simulink model "E3_QSM"  (R2025a)
settings: Solver=ode4  StartTime=0.0  StopTime=15  FixedStep=0.002  RelTol=1e-3  EnableMultiTasking=on
undefined symbols (not defined in the file): g, Jp_cm, kt, l, mode, mp, mr, nis, out_planta_e3, p, r, ref, Rm, seq, TET, tmodel, twall, Vm, xhat
libraries: simulink x6, quarc_library x4
settings Model: ExtModeTrigDuration=10000  Creator=sebas  LastModifiedBy=sebas
settings SolverCC: AlgebraicLoopSolver=TrustRegion  PositivePriorityOrder=on  EnableFixedStepZeroCrossing=on
settings DataIOCC: ReturnWorkspaceOutputs=off
settings DebuggingCC: UnconnectedInputMsg=warning  UnconnectedOutputMsg=warning  UnconnectedLineMsg=warning  ArithmeticOperatorsInVariantConditions=warning
settings HardwareCC: ProdHWDeviceType=AMD->x86-64 (Windows64)
settings ModelReferenceCC: EnableRefExpFcnMdlSchedulingChecks=on
settings SFSimCC: SimUseLocalCustomCode=off  CustomCodeUndefinedFunction=UseInterfaceOnly
settings RTWCC: SystemTargetFile=quarc_win64.tlc  TemplateMakefile=quarc_default_tmf  RTWUseLocalCustomCode=off  Toolchain=QUARC win64 | nmake (64-bit Windows)  BuildConfiguration=Faster Runs  GPUComputeCapability=3.5  Description=QUARC Win64 Target Using Toolchain
settings CodeAppCC: StateflowObjectComments=on
settings STFCustomTargetCC: SystemTargetFile=quarc_win64.tlc  TargetLangStandard=C99 (ISO)  MultiwordLength=2048.0  DynamicStringBufferSize=256.0  ConcurrentExecutionCompliant=on  UseToolchainInfoCompliant=on
settings GRTTargetCC: ExtMode=on  ExtModeMexFile=quarc_comm  ParMdlRefBuildCompliant=off  CompOptLevelCompliant=off  CombineOutputUpdateFcns=off  MatFileLogging=off  CPPClassGenCompliant=off  GRTInterface=on
settings ConfigComp: CovMetricSettings=dswe

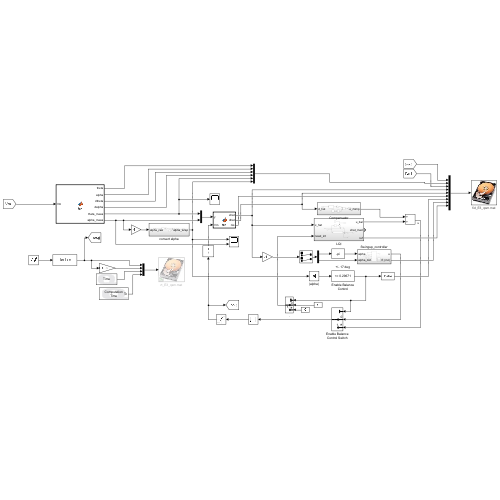
[thumbnail: Simulink's stored preview of the top-level diagram]
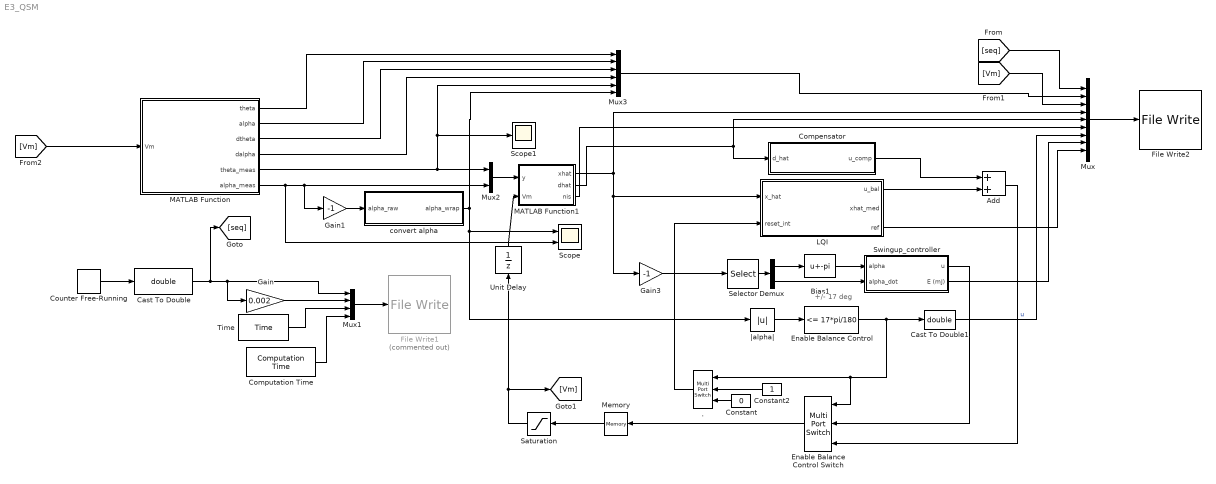
== system E3_QSM ==
  note: +/- 17 deg
  . : MultiPortSwitch  DataPortOrder=Zero-based contiguous  Inputs=2  zeroidx=on  SaturateOnIntegerOverflow=off  InputSameDT=off
  Add : Sum
  Bias1 : Bias  Bias=-pi  SaturateOnIntegerOverflow=off
  Cast To Double : DataTypeConversion  OutDataTypeStr=double  SaturateOnIntegerOverflow=off  RndMeth=Floor
  Cast To Double1 : DataTypeConversion  OutDataTypeStr=double  SaturateOnIntegerOverflow=off  RndMeth=Floor
  Compensator : Subsystem
  Computation Time : quarc_library/Sources/Time/Computation Time  sample_time=qc_get_step_size  use_model=on  use_cpu_time=off
  Constant : Constant  Value=0
  Constant2 : Constant
  Counter Free-Running : simulink/Sources/Counter Free-Running  NumBits=16  tsamp=-1
  Demux : Demux  Outputs=2
  Enable Balance Control : simulink/Logic and Bit Operations/Compare To Constant  relop=<=  const=17*pi/180  OutDataTypeStr=boolean  ZeroCross=off
  Enable Balance Control Switch : MultiPortSwitch  DataPortOrder=Zero-based contiguous  Inputs=2  zeroidx=on  SaturateOnIntegerOverflow=off  InputSameDT=off
  File Write1 : quarc_library/Sinks/To Target/File Write  Commented=on  source=Specify via dialog (do not evaluate)  file_name=rt_E3_qsm.mat  variable_name=seq,tmodel,twall,TET  decimation=1  sample_time=-1  file_format=MAT-file v.4  options=No header or footer  append=off  encoding=Default  bitrate=0
      settings: AttributesFormatString=%<file_name>  SourceProductName=QUARC Targets
  File Write2 : quarc_library/Sinks/To Target/File Write  source=Specify via dialog (do not evaluate)  file_name=fid_E3_qsm.mat  variable_name=seq,out_planta_e3,Vm,xhat.dhat,nis,mode,E,ref  decimation=1  sample_time=-1  file_format=MAT-file v.4  options=No header or footer  append=off  encoding=Default  bitrate=0
      settings: AttributesFormatString=%<file_name>  SourceProductName=QUARC Targets
  Gain : Gain  Gain=0.002
  Gain1 : Gain  Gain=-1
  Gain3 : Gain  Gain=-1
  LQI : Subsystem
  MATLAB Function : MATLAB Function  TreatAsAtomicUnit=on
  MATLAB Function1 : MATLAB Function  TreatAsAtomicUnit=on
  Memory : Memory  InheritSampleTime=on  LinearizeMemory=on  LinearizeAsDelay=on
  Mux : Mux  Inputs=9
  Mux1 : Mux
  Mux2 : Mux  Inputs=2
  Mux3 : Mux  Inputs=6
  Saturation : Saturate  UpperLimit=10  LowerLimit=-10
  Scope : Scope  NumInputPorts=2
      settings: ActiveDisplayYMinimum=-4.2429908592916838  ActiveDisplayYMaximum=6.77099119772722
  Scope1 : Scope
      settings: ActiveDisplayYMinimum=-0.93687876620115529  ActiveDisplayYMaximum=1.4676361188095872
  Selector : Selector  InputPortWidth=4  IndexOptions=Index vector (dialog)  Indices=[2 4]  OutputSizes=1
  Swingup_controller : Subsystem
  Time : quarc_library/Sources/Time/Time  time_source=Wall clock  sample_time=qc_get_step_size
  Unit Delay : UnitDelay  SampleTime=-1  HasFrameUpgradeWarning=on
  convert alpha : Subsystem
  |alpha| : Abs  SaturateOnIntegerOverflow=off
  wires:
  Computation Time/1 -> Mux1/4
  Gain/1 -> Mux1/2
  Time/1 -> Mux1/3
  Cast To Double/1 -> [seq], Mux1/1, Gain/1
  Mux1/1 -> File Write1/1
  Counter Free-Running/1 -> Cast To Double/1
  MATLAB Function1/2(dhat) -> Mux/5, Compensator/1(d_hat)
  LQI/1(u_bal) -> Add/2
  Compensator/1(u_comp) -> Add/1
  Selector/1 -> Demux/1
  |alpha|/1 -> Enable Balance Control/1
  Unit Delay/1 -> MATLAB Function1/2(Vm)
  MATLAB Function1/1(xhat) -> LQI/1(x_hat), Gain3/1, Mux/4
  Constant2/1 -> ./2
  Add/1 -> Enable Balance Control Switch/3  "u"
  Bias1/1 -> Swingup_controller/1(alpha)
  Constant/1 -> ./3
  Enable Balance Control/1 -> Cast To Double1/1, Enable Balance Control Switch/1, ./1
  Demux/2 -> Swingup_controller/2(alpha_dot)
  Demux/1 -> Bias1/1
  Swingup_controller/1(u) -> Enable Balance Control Switch/2
  Saturation/1 -> [Vm], Unit Delay/1
  Gain3/1 -> Selector/1
  ./1 -> LQI/2(reset_int)
  convert alpha/1(alpha_wrap) -> Mux3/6, |alpha|/1, Scope/1
  Mux2/1 -> MATLAB Function1/1(y)
  [seq] -> Mux/1
  MATLAB Function/3(dtheta) -> Mux3/3
  MATLAB Function/4(dalpha) -> Mux3/4
  Mux3/1 -> Mux/2
  [Vm] -> Mux/3
  MATLAB Function1/3(nis) -> Mux/6
  Swingup_controller/2(E (mJ)) -> Mux/8
  LQI/3(ref) -> Mux/9
  Mux/1 -> File Write2/1
  Cast To Double1/1 -> Mux/7
  MATLAB Function/2(alpha) -> Mux3/2
  Enable Balance Control Switch/1 -> Memory/1
  MATLAB Function/5(theta_meas) -> Mux2/1, Scope1/1, Mux3/5
  MATLAB Function/1(theta) -> Mux3/1
  [Vm] -> MATLAB Function/1(Vm)
  Memory/1 -> Saturation/1
  MATLAB Function/6(alpha_meas) -> Mux2/2, Gain1/1, Scope/2
  Gain1/1 -> convert alpha/1(alpha_raw)

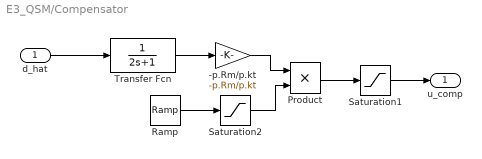
== system E3_QSM/Compensator ==
  d_hat : Inport
  -p.Rm/p.kt : Gain  Gain=-p.Rm/p.kt
  Product : Product
  Ramp : simulink/Sources/Ramp  slope=0.5  start=0  InitialOutput=0
  Saturation1 : Saturate  UpperLimit=2  LowerLimit=-2
  Saturation2 : Saturate  UpperLimit=1  LowerLimit=0
  Transfer Fcn : TransferFcn  Denominator=[2 1]
  u_comp : Outport
  wires:
  Saturation1/1 -> u_comp/1
  Transfer Fcn/1 -> -p.Rm/p.kt/1
  -p.Rm/p.kt/1 -> Product/1
  Saturation2/1 -> Product/2
  Ramp/1 -> Saturation2/1
  d_hat/1 -> Transfer Fcn/1
  Product/1 -> Saturation1/1

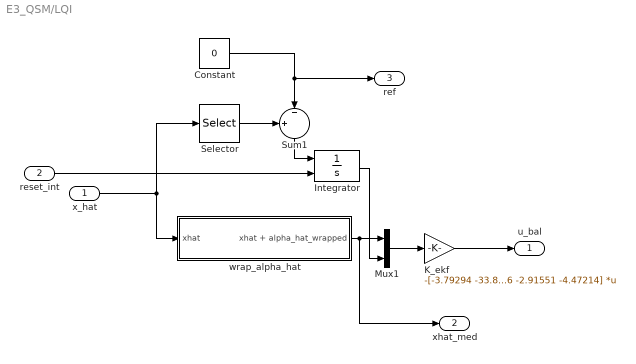
== system E3_QSM/LQI ==
  x_hat : Inport
  reset_int : Inport  Port=2
  Constant : Constant  Value=0
  Integrator : Integrator  ExternalReset=level hold  LimitOutput=on  UpperSaturationLimit=2  LowerSaturationLimit=-2
  K_ekf : Gain  Gain=-[-3.79294 -33.8988 -1.48036 -2.91551 -4.47214]  Multiplication=Matrix(K*u)
  Mux1 : Mux  Inputs=2
  Selector : Selector  InputPortWidth=4  IndexOptions=Index vector (dialog)  Indices=[1]  OutputSizes=1
  Sum1 : Sum  Inputs=+|-||
  wrap_alpha_hat : Subsystem
  u_bal : Outport
  xhat_med : Outport  Port=2
  ref : Outport  Port=3
  wires:
  Integrator/1 -> Mux1/2
  Mux1/1 -> K_ekf/1
  Constant/1 -> ref/1, Sum1/2
  Sum1/1 -> Integrator/1
  Selector/1 -> Sum1/1
  K_ekf/1 -> u_bal/1
  reset_int/1 -> Integrator/2
  x_hat/1 -> wrap_alpha_hat/1(xhat), Selector/1
  wrap_alpha_hat/1(xhat + alpha_hat_wrapped) -> xhat_med/1, Mux1/1

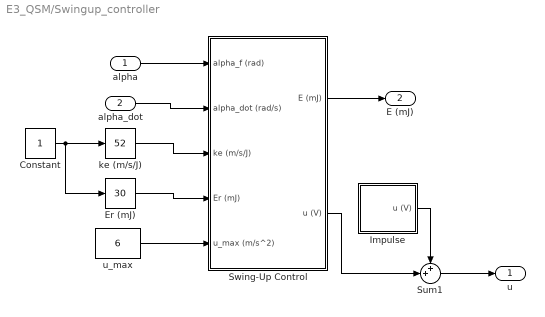
== system E3_QSM/Swingup_controller ==
  alpha : Inport
  alpha_dot : Inport  Port=2
  Constant : Constant
  Er (mJ) : simulink/Math Operations/Slider Gain  gain=30  low=0  high=100
  Impulse : Subsystem
  Sum1 : Sum  Inputs=++|
  Swing-Up Control : Subsystem
  ke (m/s/J) : simulink/Math Operations/Slider Gain  gain=52  low=0  high=100
  u_max : Constant  Value=6
  u : Outport
  E (mJ) : Outport  Port=2
  wires:
  alpha/1 -> Swing-Up Control/1(alpha_f (rad))
  Sum1/1 -> u/1
  u_max/1 -> Swing-Up Control/5(u_max (m/s^2))
  Impulse/1(u (V)) -> Sum1/1
  Swing-Up Control/1(E (mJ)) -> E (mJ)/1
  Swing-Up Control/2(u (V)) -> Sum1/2
  ke (m/s/J)/1 -> Swing-Up Control/3(ke (m/s/J))
  Constant/1 -> Er (mJ)/1, ke (m/s/J)/1
  Er (mJ)/1 -> Swing-Up Control/4(Er (mJ))
  alpha_dot/1 -> Swing-Up Control/2(alpha_dot (rad/s))

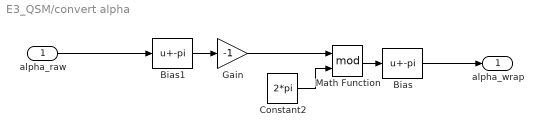
== system E3_QSM/convert alpha ==
  alpha_raw : Inport
  Bias : Bias  Bias=-pi  SaturateOnIntegerOverflow=off
  Bias1 : Bias  Bias=-pi  SaturateOnIntegerOverflow=off
  Constant2 : Constant  Value=2*pi
  Gain : Gain  Gain=-1
  Math Function : Math  Operator=mod  SignedPower=on
  alpha_wrap : Outport
  wires:
  Math Function/1 -> Bias/1
  Bias/1 -> alpha_wrap/1
  Constant2/1 -> Math Function/2
  alpha_raw/1 -> Bias1/1
  Bias1/1 -> Gain/1
  Gain/1 -> Math Function/1

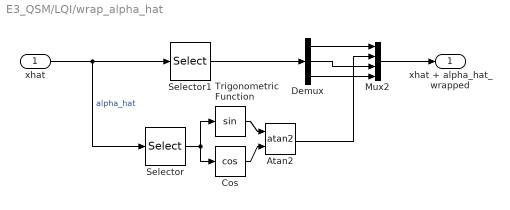
== system E3_QSM/LQI/wrap_alpha_hat ==
  xhat : Inport
  Atan2 : Trigonometry  Operator=atan2
  Cos : Trigonometry  Operator=cos
  Demux : Demux  Outputs=3
  Mux2 : Mux
  Selector : Selector  InputPortWidth=4  IndexOptions=Index vector (dialog)  Indices=[2]  OutputSizes=1
  Selector1 : Selector  InputPortWidth=4  IndexOptions=Index vector (dialog)  Indices=[1 3 4]  OutputSizes=1
  Trigonometric Function : Trigonometry
  xhat + alpha_hat_wrapped : Outport
  wires:
  Selector/1 -> Cos/1, Trigonometric Function/1
  Mux2/1 -> xhat + alpha_hat_wrapped/1
  Cos/1 -> Atan2/2
  xhat/1 -> Selector/1, Selector1/1  "alpha_hat"
  Trigonometric Function/1 -> Atan2/1
  Demux/2 -> Mux2/3
  Selector1/1 -> Demux/1
  Demux/1 -> Mux2/1
  Demux/3 -> Mux2/4
  Atan2/1 -> Mux2/2

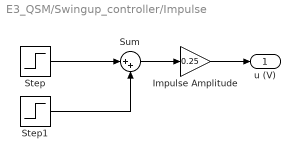
== system E3_QSM/Swingup_controller/Impulse ==
  Impulse Amplitude : Gain  Gain=0.25
  Step : Step  SampleTime=0
  Step1 : Step  Time=1.1  After=-1  SampleTime=0
  Sum : Sum  Inputs=|++
  u (V) : Outport  VectorParamsAs1DForOutWhenUnconnected=off
  wires:
  Impulse Amplitude/1 -> u (V)/1
  Sum/1 -> Impulse Amplitude/1
  Step/1 -> Sum/1
  Step1/1 -> Sum/2

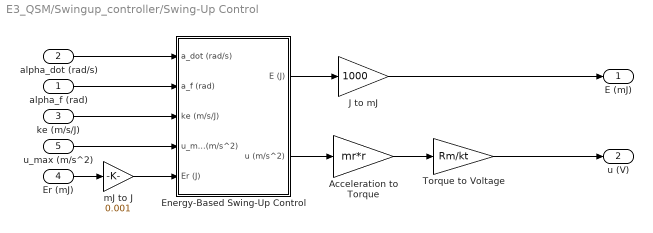
== system E3_QSM/Swingup_controller/Swing-Up Control ==
  alpha_f (rad) : Inport
  alpha_dot (rad/s) : Inport  Port=2
  ke (m/s/J) : Inport  Port=3
  Er (mJ) : Inport  Port=4
  u_max (m/s^2) : Inport  Port=5
  Acceleration to Torque : Gain  Gain=mr*r
  Energy-Based Swing-Up Control : Subsystem
  J to mJ : Gain  Gain=1000
  Torque to Voltage : Gain  Gain=Rm/kt
  mJ to J : Gain  Gain=0.001
  E (mJ) : Outport  VectorParamsAs1DForOutWhenUnconnected=off
  u (V) : Outport  Port=2  VectorParamsAs1DForOutWhenUnconnected=off
  wires:
  mJ to J/1 -> Energy-Based Swing-Up Control/5(Er (J))
  alpha_dot (rad/s)/1 -> Energy-Based Swing-Up Control/1(a_dot (rad/s))
  Torque to Voltage/1 -> u (V)/1
  J to mJ/1 -> E (mJ)/1
  Er (mJ)/1 -> mJ to J/1
  Acceleration to Torque/1 -> Torque to Voltage/1
  u_max (m/s^2)/1 -> Energy-Based Swing-Up Control/4(u_max (m/s^2))
  ke (m/s/J)/1 -> Energy-Based Swing-Up Control/3(ke (m/s/J))
  alpha_f (rad)/1 -> Energy-Based Swing-Up Control/2(a_f (rad))
  Energy-Based Swing-Up Control/1(E (J)) -> J to mJ/1
  Energy-Based Swing-Up Control/2(u (m/s^2)) -> Acceleration to Torque/1

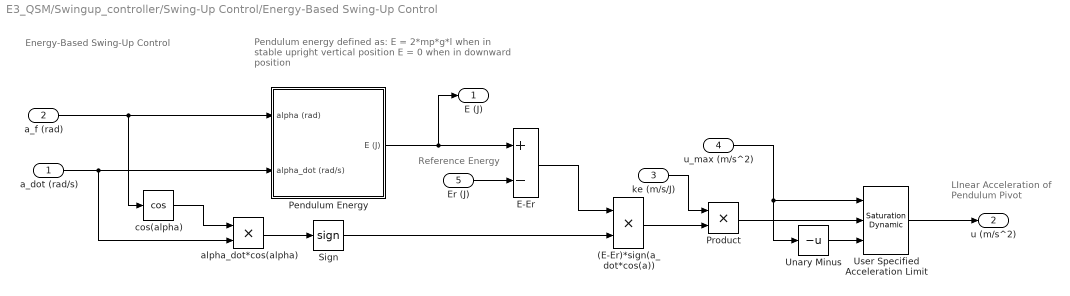
== system E3_QSM/Swingup_controller/Swing-Up Control/Energy-Based Swing-Up Control ==
  note: Pendulum energy defined as:
      | E = 2*mp*g*l when in stable upright vertical position
      | E = 0 when in downward position
  note: Reference Energy
  note: LInear Acceleration of
      | Pendulum Pivot
  note: Energy-Based Swing-Up Control
  a_dot (rad/s) : Inport
  a_f (rad) : Inport  Port=2
  ke (m/s/J) : Inport  Port=3
  u_max (m/s^2) : Inport  Port=4
  Er (J) : Inport  Port=5
  (E-Er)*sign(a_dot*cos(a)) : Product  RndMeth=Zero
  E-Er : Sum  Inputs=+-
  Pendulum Energy : Subsystem
  Product : Product  RndMeth=Zero
  Sign : Signum
  Unary Minus : UnaryMinus
  User Specified Acceleration Limit : simulink/Discontinuities/Saturation Dynamic  OutMin=[]  OutMax=[]  OutDataTypeStr=Inherit: Same as second input  OutDataType=fixdt(1, 16)  OutScaling=2^-10  DoSatur=off
  alpha_dot*cos(alpha) : Product  RndMeth=Zero
  cos(alpha) : Trigonometry  Operator=cos
  E (J) : Outport  VectorParamsAs1DForOutWhenUnconnected=off
  u (m/s^2) : Outport  Port=2  VectorParamsAs1DForOutWhenUnconnected=off
  wires:
  User Specified Acceleration Limit/1 -> u (m/s^2)/1
  Unary Minus/1 -> User Specified Acceleration Limit/3
  u_max (m/s^2)/1 -> Unary Minus/1, User Specified Acceleration Limit/1
  Product/1 -> User Specified Acceleration Limit/2
  ke (m/s/J)/1 -> Product/1
  Er (J)/1 -> E-Er/2
  (E-Er)*sign(a_dot*cos(a))/1 -> Product/2
  a_dot (rad/s)/1 -> Pendulum Energy/2(alpha_dot (rad/s)), alpha_dot*cos(alpha)/2
  Pendulum Energy/1(E (J)) -> E-Er/1, E (J)/1
  E-Er/1 -> (E-Er)*sign(a_dot*cos(a))/1
  cos(alpha)/1 -> alpha_dot*cos(alpha)/1
  alpha_dot*cos(alpha)/1 -> Sign/1
  Sign/1 -> (E-Er)*sign(a_dot*cos(a))/2
  a_f (rad)/1 -> cos(alpha)/1, Pendulum Energy/1(alpha (rad))

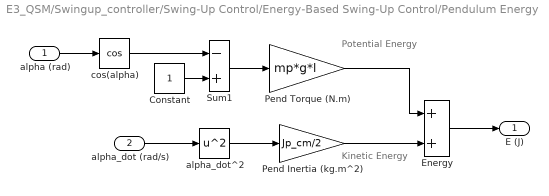
== system E3_QSM/Swingup_controller/Swing-Up Control/Energy-Based Swing-Up Control/Pendulum Energy ==
  note: Potential Energy
  note: Kinetic Energy
  alpha (rad) : Inport
  alpha_dot (rad/s) : Inport  Port=2
  Constant : Constant
  Energy : Sum  SaturateOnIntegerOverflow=on
  Pend Inertia (kg.m^2) : Gain  Gain=Jp_cm/2
  Pend Torque (N.m) : Gain  Gain=mp*g*l
  Sum1 : Sum  Inputs=-+  SaturateOnIntegerOverflow=on
  alpha_dot^2 : Math  Operator=square  SignedPower=on
  cos(alpha) : Trigonometry  Operator=cos
  E (J) : Outport  VectorParamsAs1DForOutWhenUnconnected=off
  wires:
  cos(alpha)/1 -> Sum1/1
  Energy/1 -> E (J)/1
  alpha_dot (rad/s)/1 -> alpha_dot^2/1
  alpha (rad)/1 -> cos(alpha)/1
  Pend Torque (N.m)/1 -> Energy/1
  alpha_dot^2/1 -> Pend Inertia (kg.m^2)/1
  Pend Inertia (kg.m^2)/1 -> Energy/2
  Constant/1 -> Sum1/2
  Sum1/1 -> Pend Torque (N.m)/1

== matlab function E3_QSM/MATLAB Function1 ==
  data: y input; xhat output; Vm input; dhat output; nis output size=1
function [xhat, dhat,nis] = fcn(y, Vm)
   [xhat, dhat,nis] = ekf_step(y, Vm);
end

== matlab function E3_QSM/MATLAB Function ==
  data: Vm input; theta output; alpha output; dtheta output; dalpha output; theta_meas output; alpha_meas output
function [theta,alpha,dtheta,dalpha,theta_meas,alpha_meas] = fcn(Vm)
%#codegen
% E1: x0=[0;0.05;0;0]  |  E2 y E3: x0=[0;pi;0;0]
[theta,alpha,dtheta,dalpha,theta_meas,alpha_meas] = ...
    furuta_planta_analitica(Vm, [0;pi;0;0], 0.002, 8);
end
